simulink model "DiscreteControllerSim"  (R2015b)
settings: Solver=VariableStepAuto  StartTime=0.0  StopTime=t  RelTol=1e-3
values from neighbouring files (symbols this model uses):
  A12 = A(1:3,4:6)    [StateSpace.m]
  C_x = 0.55    [DiscreteController.m]
  C_xdot = -0.17    [DiscreteController.m]
  C_y = 0.55    [DiscreteController.m]
  C_ydot = 0.17    [DiscreteController.m]
  C_z = 0.9    [DiscreteController.m]
  Lobs = (-place(A22',A12',[-20 -25 -30]))'    [StateSpace.m]
  step_x = 1    [DiscreteController.m]
  T = 0.035    [DiscreteController.m]
  x_ref = 1    [plotSim.m]
  x_ref_time = 0.1    [plotSim.m]
  y_ref = 1    [plotSim.m]
  y_ref_time = 5    [plotSim.m]
  z_ref = 1    [plotSim.m]
  z_ref_time = 10    [plotSim.m]
undefined symbols (not defined in the file or in its folder): Fg, Jx, Jy, Jz, kd, kth, L, m, w1_bar, w2_bar, w3_bar, w4_bar
settings Model: Creator=USUARIO  LastModifiedBy=USUARIO

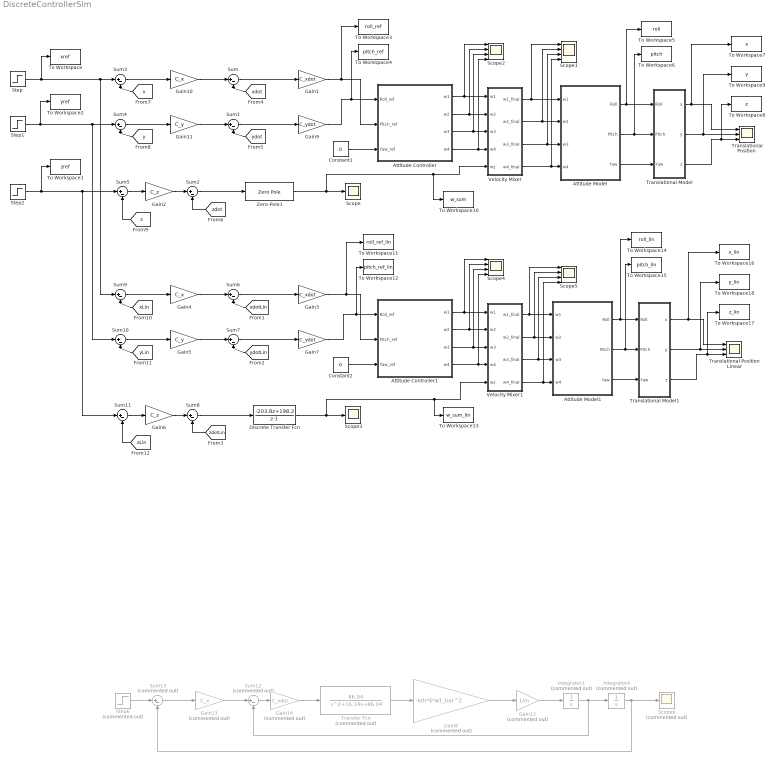
== system DiscreteControllerSim ==
  Attitude Controller : Subsystem
  Attitude Controller1 : Subsystem
  Attitude Model : Subsystem
  Attitude Model1 : Subsystem
  Constant1 : Constant  Value=0
  Constant2 : Constant  Value=0
  Discrete Transfer Fcn : DiscreteTransferFcn  Numerator=[-203.8 198.2]  Denominator=[1 -1]  SampleTime=T
  Gain1 : Gain  Gain=C_xdot
  Gain10 : Gain  Gain=C_x
  Gain11 : Gain  Gain=C_y
  Gain12 : Gain  Commented=on  Gain=1/m
  Gain13 : Gain  Commented=on  Gain=C_x
  Gain14 : Gain  Commented=on  Gain=C_xdot
  Gain2 : Gain  Gain=C_z
  Gain3 : Gain  Gain=C_xdot
  Gain4 : Gain  Gain=C_x
  Gain5 : Gain  Gain=C_y
  Gain6 : Gain  Gain=C_z
  Gain7 : Gain  Gain=C_ydot
  Gain8 : Gain  Commented=on  Gain=-kth*4*w1_bar^2
  Gain9 : Gain  Gain=C_ydot
  Integrator1 : Integrator  Commented=on
  Integrator4 : Integrator  Commented=on
  Scope : Scope
  Scope{1..2,4..5} (4 alike) : Scope  NumInputPorts=4
  Scope3 : Scope
  Scope6 : Scope  Commented=on
  Step : Step  Time=x_ref_time  After=x_ref  SampleTime=0
  Step1 : Step  Time=y_ref_time  After=y_ref  SampleTime=0
  Step2 : Step  Time=z_ref_time  After=z_ref  SampleTime=0
  Step6 : Step  Commented=on  Time=0  After=step_x  SampleTime=0
  Sum{,1..11} (12 alike) : Sum  Inputs=|+-
  Sum12 : Sum  Commented=on  Inputs=|+-
  Sum13 : Sum  Commented=on  Inputs=|+-
  To Workspace : ToWorkspace  VariableName=xref  SaveFormat=Timeseries  SampleTime=-1
  To Workspace1 : ToWorkspace  VariableName=zref  SaveFormat=Timeseries  SampleTime=-1
  To Workspace10 : ToWorkspace  VariableName=w_sum  SaveFormat=Timeseries  SampleTime=-1
  To Workspace11 : ToWorkspace  VariableName=roll_ref_lin  SaveFormat=Timeseries  SampleTime=-1
  To Workspace12 : ToWorkspace  VariableName=pitch_ref_lin  SaveFormat=Timeseries  SampleTime=-1
  To Workspace13 : ToWorkspace  VariableName=w_sum_lin  SaveFormat=Timeseries  SampleTime=-1
  To Workspace14 : ToWorkspace  VariableName=roll_lin  SaveFormat=Timeseries  SampleTime=-1
  To Workspace15 : ToWorkspace  VariableName=pitch_lin  SaveFormat=Timeseries  SampleTime=-1
  To Workspace16 : ToWorkspace  VariableName=x_lin  SaveFormat=Timeseries  SampleTime=-1
  To Workspace17 : ToWorkspace  VariableName=z_lin  SaveFormat=Timeseries  SampleTime=-1
  To Workspace18 : ToWorkspace  VariableName=y_lin  SaveFormat=Timeseries  SampleTime=-1
  To Workspace2 : ToWorkspace  VariableName=yref  SaveFormat=Timeseries  SampleTime=-1
  To Workspace3 : ToWorkspace  VariableName=roll_ref  SaveFormat=Timeseries  SampleTime=-1
  To Workspace4 : ToWorkspace  VariableName=pitch_ref  SaveFormat=Timeseries  SampleTime=-1
  To Workspace5 : ToWorkspace  VariableName=roll  SaveFormat=Timeseries  SampleTime=-1
  To Workspace6 : ToWorkspace  VariableName=pitch  SaveFormat=Timeseries  SampleTime=-1
  To Workspace7 : ToWorkspace  VariableName=x  SaveFormat=Timeseries  SampleTime=-1
  To Workspace8 : ToWorkspace  VariableName=z  SaveFormat=Timeseries  SampleTime=-1
  To Workspace9 : ToWorkspace  VariableName=y  SaveFormat=Timeseries  SampleTime=-1
  Transfer Fcn : TransferFcn  Commented=on  Numerator=[86.04]  Denominator=[1 16.14 86.04]
  Translational Position : Scope  NumInputPorts=3
  Translational Position Linear : Scope  NumInputPorts=3
  Translational Model : Subsystem
  Translational Model1 : Subsystem
  Velocity Mixer : Subsystem
  Velocity Mixer1 : Subsystem
  Zero-Pole1 : ZeroPole  Zeros=[-0.8]  Poles=[0]  Gain=[-200]
  wires:
  Sum/1 -> Gain1/1
  Sum1/1 -> Gain9/1
  Sum2/1 -> Zero-Pole1/1
  [zdot] -> Sum2/2
  [ydot] -> Sum1/2
  [xdot] -> Sum/2
  Gain10/1 -> Sum/1
  Gain11/1 -> Sum1/1
  Constant1/1 -> Attitude Controller/3(Yaw_ref)
  Gain1/1 -> To Workspace3/1, Attitude Controller/2(Pitch_ref)
  Gain9/1 -> To Workspace4/1, Attitude Controller/1(Roll_ref)
  Velocity Mixer/1(w1_final) -> Scope1/1, Attitude Model/1(w1)
  Velocity Mixer/2(w2_final) -> Scope1/2, Attitude Model/2(w2)
  Velocity Mixer/3(w3_final) -> Scope1/3, Attitude Model/3(w3)
  Velocity Mixer/4(w4_final) -> Scope1/4, Attitude Model/4(w4)
  Zero-Pole1/1 -> To Workspace10/1, Velocity Mixer/5(wz), Scope/1
  Attitude Controller/1(w1) -> Velocity Mixer/1(w1), Scope2/1
  Attitude Controller/2(w2) -> Velocity Mixer/2(w2), Scope2/2
  Attitude Controller/3(w3) -> Velocity Mixer/3(w3), Scope2/3
  Attitude Controller/4(w4) -> Velocity Mixer/4(w4), Scope2/4
  Gain2/1 -> Sum2/1
  Attitude Model/1(Roll) -> To Workspace5/1, Translational Model/1(Roll)
  Translational Model/1(x) -> To Workspace7/1, Translational Position/1
  Translational Model/2(y) -> To Workspace9/1, Translational Position/2
  Translational Model/3(z) -> To Workspace8/1, Translational Position/3
  Attitude Model/2(Pitch) -> To Workspace6/1, Translational Model/2(Pitch)
  Sum3/1 -> Gain10/1
  Sum4/1 -> Gain11/1
  [y] -> Sum4/2
  [x] -> Sum3/2
  [z] -> Sum5/2
  Sum5/1 -> Gain2/1
  Attitude Model/3(Yaw) -> Translational Model/3("Yaw ")
  Attitude Model1/1(Roll) -> To Workspace14/1, Translational Model1/1(Roll)
  Translational Model1/1(x) -> To Workspace16/1, Translational Position Linear/1
  Translational Model1/2(y) -> To Workspace18/1, Translational Position Linear/2
  Translational Model1/3(z) -> To Workspace17/1, Translational Position Linear/3
  Sum6/1 -> Gain3/1
  Sum7/1 -> Gain7/1
  Sum8/1 -> Discrete Transfer Fcn/1
  [zdotLin] -> Sum8/2
  [ydotLin] -> Sum7/2
  [xdotLin] -> Sum6/2
  Gain4/1 -> Sum6/1
  Gain5/1 -> Sum7/1
  Constant2/1 -> Attitude Controller1/3(Yaw_ref)
  Attitude Controller1/1(w1) -> Velocity Mixer1/1(w1), Scope4/1
  Attitude Controller1/2(w2) -> Velocity Mixer1/2(w2), Scope4/2
  Attitude Controller1/3(w3) -> Velocity Mixer1/3(w3), Scope4/3
  Attitude Controller1/4(w4) -> Velocity Mixer1/4(w4), Scope4/4
  Gain6/1 -> Sum8/1
  Sum9/1 -> Gain4/1
  Sum10/1 -> Gain5/1
  [yLin] -> Sum10/2
  [xLin] -> Sum9/2
  [zLin] -> Sum11/2
  Step2/1 -> To Workspace1/1, Sum11/1, Sum5/1
  Sum11/1 -> Gain6/1
  Step/1 -> To Workspace/1, Sum9/1, Sum3/1
  Step1/1 -> To Workspace2/1, Sum10/1, Sum4/1
  Velocity Mixer1/1(w1_final) -> Scope5/1, Attitude Model1/1(w1)
  Velocity Mixer1/2(w2_final) -> Scope5/2, Attitude Model1/2(w2)
  Velocity Mixer1/3(w3_final) -> Scope5/3, Attitude Model1/3(w3)
  Velocity Mixer1/4(w4_final) -> Scope5/4, Attitude Model1/4(w4)
  Transfer Fcn/1 -> Gain8/1
  Gain8/1 -> Gain12/1
  Gain12/1 -> Integrator1/1
  Sum12/1 -> Gain14/1
  Integrator1/1 -> Sum12/2, Integrator4/1
  Gain13/1 -> Sum12/1
  Sum13/1 -> Gain13/1
  Integrator4/1 -> Scope6/1, Sum13/2
  Step6/1 -> Sum13/1
  Gain14/1 -> Transfer Fcn/1
  Gain3/1 -> To Workspace11/1, Attitude Controller1/2(Pitch_ref)
  Gain7/1 -> To Workspace12/1, Attitude Controller1/1(Roll_ref)
  Discrete Transfer Fcn/1 -> Velocity Mixer1/5(wz), To Workspace13/1, Scope3/1
  Attitude Model1/2(Pitch) -> To Workspace15/1, Translational Model1/2(Pitch)
  Attitude Model1/3(Yaw) -> Translational Model1/3(Yaw)

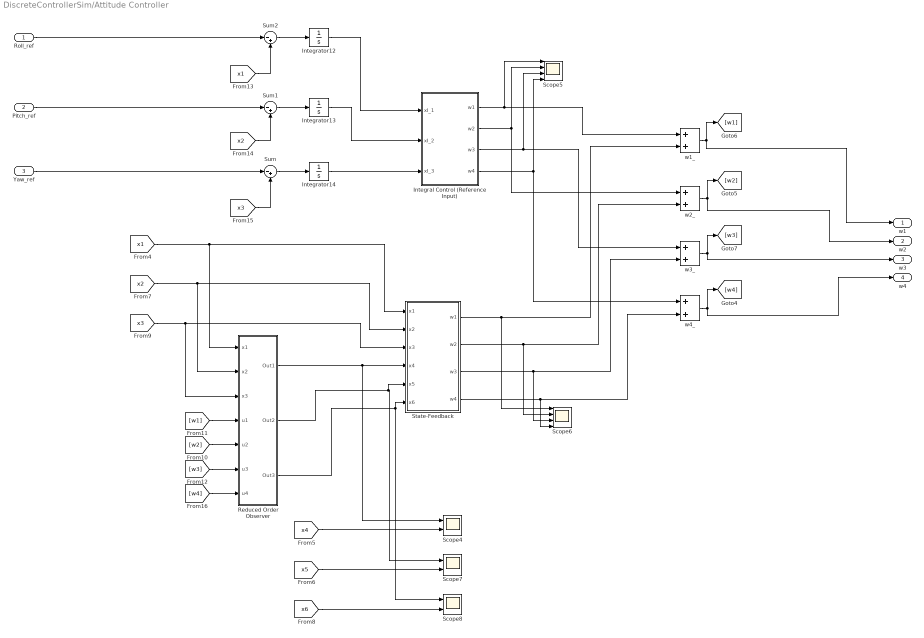
== system DiscreteControllerSim/Attitude Controller ==
  Roll_ref : Inport
  Pitch_ref : Inport  Port=2
  Yaw_ref : Inport  Port=3
  Integral Control (Reference Input) : MATLAB Function  TreatAsAtomicUnit=on
  Integrator12 : Integrator
  Integrator13 : Integrator
  Integrator14 : Integrator
  Reduced Order Observer : Subsystem
  Scope4 : Scope  NumInputPorts=2
  Scope5 : Scope  NumInputPorts=4
  Scope6 : Scope  NumInputPorts=4
  Scope7 : Scope  NumInputPorts=2
  Scope8 : Scope  NumInputPorts=2
  "State-Feedback " : MATLAB Function  TreatAsAtomicUnit=on
  Sum : Sum  Inputs=|-+
  Sum1 : Sum  Inputs=|-+
  Sum2 : Sum  Inputs=|-+
  w1_ : Sum
  w2_ : Sum
  w3_ : Sum
  w4_ : Sum
  w1 : Outport
  w2 : Outport  Port=2
  w3 : Outport  Port=3
  w4 : Outport  Port=4
  wires:
  "State-Feedback "/4(w4) -> w4_/2, Scope6/4
  Roll_ref/1 -> Sum2/1
  [x3] -> Sum/2
  [x1] -> Sum2/2
  Integrator13/1 -> Integral Control (Reference Input)/2(xI_2)
  "State-Feedback "/1(w1) -> w1_/2, Scope6/1
  [w3] -> Reduced Order Observer/6(u3)
  Sum2/1 -> Integrator12/1
  Sum/1 -> Integrator14/1
  [x3] -> "State-Feedback "/3(x3), Reduced Order Observer/3(x3)
  [w2] -> Reduced Order Observer/5(u2)
  Pitch_ref/1 -> Sum1/1
  Integrator14/1 -> Integral Control (Reference Input)/3(xI_3)
  Reduced Order Observer/3(Out3) -> "State-Feedback "/6(x6), Scope8/1
  [x4] -> Scope4/2
  [x6] -> Scope8/2
  "State-Feedback "/2(w2) -> w2_/2, Scope6/2
  Integral Control (Reference Input)/2(w2) -> Scope5/2, w2_/1
  [w4] -> Reduced Order Observer/7(u4)
  Integral Control (Reference Input)/3(w3) -> w3_/1, Scope5/3
  Reduced Order Observer/2(Out2) -> "State-Feedback "/5(x5), Scope7/1
  [x1] -> "State-Feedback "/1(x1), Reduced Order Observer/1(x1)
  [w1] -> Reduced Order Observer/4(u1)
  Integrator12/1 -> Integral Control (Reference Input)/1(xI_1)
  [x2] -> Sum1/2
  Integral Control (Reference Input)/4(w4) -> Scope5/4, w4_/1
  Integral Control (Reference Input)/1(w1) -> w1_/1, Scope5/1
  [x2] -> "State-Feedback "/2(x2), Reduced Order Observer/2(x2)
  Reduced Order Observer/1(Out1) -> "State-Feedback "/4(x4), Scope4/1
  [x5] -> Scope7/2
  Sum1/1 -> Integrator13/1
  Yaw_ref/1 -> Sum/1
  "State-Feedback "/3(w3) -> w3_/2, Scope6/3
  w1_/1 -> w1/1, [w1]
  w4_/1 -> w4/1, [w4]
  w2_/1 -> w2/1, [w2]
  w3_/1 -> w3/1, [w3]

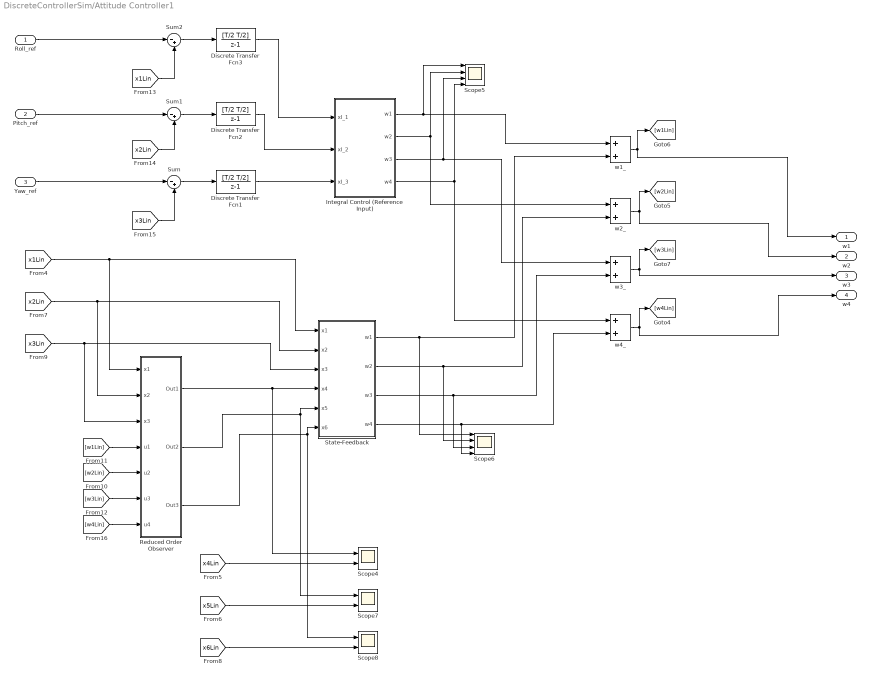
== system DiscreteControllerSim/Attitude Controller1 ==
  Roll_ref : Inport
  Pitch_ref : Inport  Port=2
  Yaw_ref : Inport  Port=3
  Discrete Transfer Fcn1 : DiscreteTransferFcn  Numerator=[T/2 T/2]  Denominator=[1 -1]  SampleTime=T
  Discrete Transfer Fcn2 : DiscreteTransferFcn  Numerator=[T/2 T/2]  Denominator=[1 -1]  SampleTime=T
  Discrete Transfer Fcn3 : DiscreteTransferFcn  Numerator=[T/2 T/2]  Denominator=[1 -1]  SampleTime=T
  Integral Control (Reference Input) : MATLAB Function  TreatAsAtomicUnit=on
  Reduced Order Observer : Subsystem
  Scope4 : Scope  NumInputPorts=2
  Scope5 : Scope  NumInputPorts=4
  Scope6 : Scope  NumInputPorts=4
  Scope7 : Scope  NumInputPorts=2
  Scope8 : Scope  NumInputPorts=2
  "State-Feedback " : MATLAB Function  TreatAsAtomicUnit=on
  Sum : Sum  Inputs=|-+
  Sum1 : Sum  Inputs=|-+
  Sum2 : Sum  Inputs=|-+
  w1_ : Sum
  w2_ : Sum
  w3_ : Sum
  w4_ : Sum
  w1 : Outport
  w2 : Outport  Port=2
  w3 : Outport  Port=3
  w4 : Outport  Port=4
  wires:
  "State-Feedback "/4(w4) -> w4_/2, Scope6/4
  Roll_ref/1 -> Sum2/1
  [x3Lin] -> Sum/2
  [x1Lin] -> Sum2/2
  Discrete Transfer Fcn2/1 -> Integral Control (Reference Input)/2(xI_2)
  "State-Feedback "/1(w1) -> w1_/2, Scope6/1
  [w3Lin] -> Reduced Order Observer/6(u3)
  Sum2/1 -> Discrete Transfer Fcn3/1
  Sum/1 -> Discrete Transfer Fcn1/1
  [x3Lin] -> "State-Feedback "/3(x3), Reduced Order Observer/3(x3)
  [w2Lin] -> Reduced Order Observer/5(u2)
  Pitch_ref/1 -> Sum1/1
  Discrete Transfer Fcn1/1 -> Integral Control (Reference Input)/3(xI_3)
  Reduced Order Observer/3(Out3) -> "State-Feedback "/6(x6), Scope8/1
  [x4Lin] -> Scope4/2
  [x6Lin] -> Scope8/2
  "State-Feedback "/2(w2) -> w2_/2, Scope6/2
  Integral Control (Reference Input)/2(w2) -> Scope5/2, w2_/1
  [w4Lin] -> Reduced Order Observer/7(u4)
  Integral Control (Reference Input)/3(w3) -> w3_/1, Scope5/3
  Reduced Order Observer/2(Out2) -> "State-Feedback "/5(x5), Scope7/1
  [x1Lin] -> "State-Feedback "/1(x1), Reduced Order Observer/1(x1)
  [w1Lin] -> Reduced Order Observer/4(u1)
  Discrete Transfer Fcn3/1 -> Integral Control (Reference Input)/1(xI_1)
  [x2Lin] -> Sum1/2
  Integral Control (Reference Input)/4(w4) -> Scope5/4, w4_/1
  Integral Control (Reference Input)/1(w1) -> w1_/1, Scope5/1
  [x2Lin] -> "State-Feedback "/2(x2), Reduced Order Observer/2(x2)
  Reduced Order Observer/1(Out1) -> "State-Feedback "/4(x4), Scope4/1
  [x5Lin] -> Scope7/2
  Sum1/1 -> Discrete Transfer Fcn2/1
  Yaw_ref/1 -> Sum/1
  "State-Feedback "/3(w3) -> w3_/2, Scope6/3
  w1_/1 -> w1/1, [w1Lin]
  w4_/1 -> w4/1, [w4Lin]
  w2_/1 -> w2/1, [w2Lin]
  w3_/1 -> w3/1, [w3Lin]

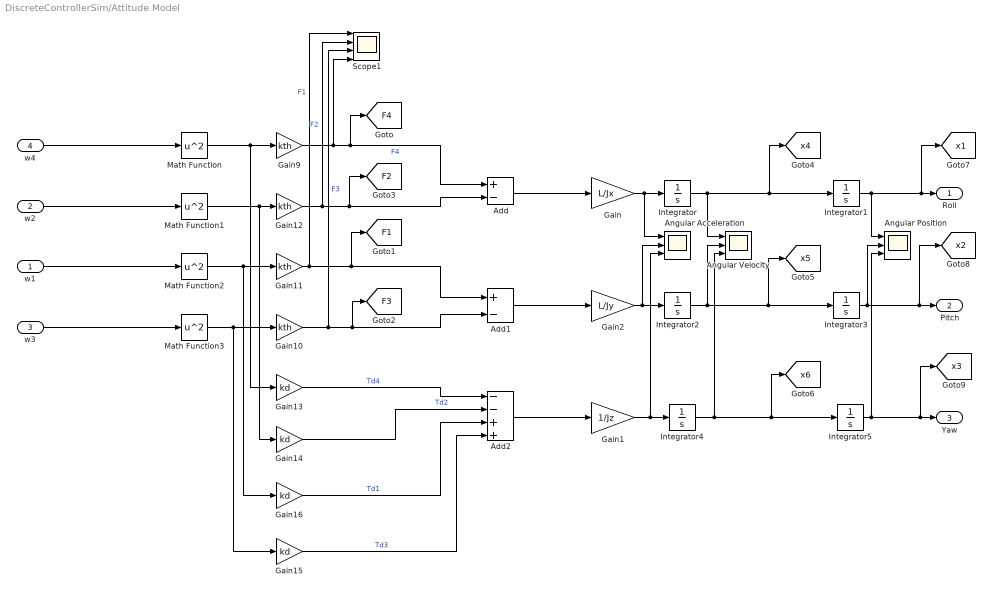
== system DiscreteControllerSim/Attitude Model ==
  w1 : Inport
  w2 : Inport  Port=2
  w3 : Inport  Port=3
  w4 : Inport  Port=4
  Add : Sum  Inputs=+-
  Add1 : Sum  Inputs=+-
  Add2 : Sum  Inputs=--++
  Angular Position : Scope  NumInputPorts=3
  Angular Velocity : Scope  NumInputPorts=3
  Angular Acceleration : Scope  NumInputPorts=3
  Gain : Gain  Gain=L/Jx
  Gain1 : Gain  Gain=1/Jz
  Gain{9..12} (4 alike) : Gain  Gain=kth
  Gain{13..16} (4 alike) : Gain  Gain=kd
  Gain2 : Gain  Gain=L/Jy
  Integrator{,1..5} (6 alike) : Integrator
  Math Function{,1..3} (4 alike) : Math  Operator=square  SaturateOnIntegerOverflow=on
  Scope1 : Scope  NumInputPorts=4
  Roll : Outport
  Pitch : Outport  Port=2
  Yaw : Outport  Port=3
  tag scope: F1=global, F2=global, F3=global, F4=global, x1=global, x2=global, x3=global, x4=global, x5=global, x6=global
  wires:
  Gain2/1 -> Angular Acceleration/2, Integrator2/1
  Add2/1 -> Gain1/1
  Gain9/1 -> Scope1/4, [F4], Add/1  "F4"
  Gain14/1 -> Add2/2  "Td2"
  Gain16/1 -> Add2/3  "Td1"
  Gain/1 -> Angular Acceleration/1, Integrator/1
  Integrator/1 -> Angular Velocity/1, Integrator1/1, [x4]
  Integrator1/1 -> [x1], Roll/1, Angular Position/1
  Integrator4/1 -> Angular Velocity/3, [x6], Integrator5/1
  Add/1 -> Gain/1
  Integrator3/1 -> [x2], Pitch/1, Angular Position/2
  Add1/1 -> Gain2/1
  Integrator5/1 -> Angular Position/3, [x3], Yaw/1
  Gain12/1 -> Scope1/2, [F2], Add/2  "F2"
  Gain10/1 -> [F3], Add1/2, Scope1/3  "F3"
  Gain11/1 -> Scope1/1, [F1], Add1/1  "F1"
  Gain13/1 -> Add2/1  "Td4"
  Gain15/1 -> Add2/4  "Td3"
  Integrator2/1 -> Angular Velocity/2, [x5], Integrator3/1
  Gain1/1 -> Angular Acceleration/3, Integrator4/1
  Math Function3/1 -> Gain15/1, Gain10/1
  Math Function2/1 -> Gain16/1, Gain11/1
  Math Function/1 -> Gain13/1, Gain9/1
  Math Function1/1 -> Gain14/1, Gain12/1
  w1/1 -> Math Function2/1
  w2/1 -> Math Function1/1
  w3/1 -> Math Function3/1
  w4/1 -> Math Function/1

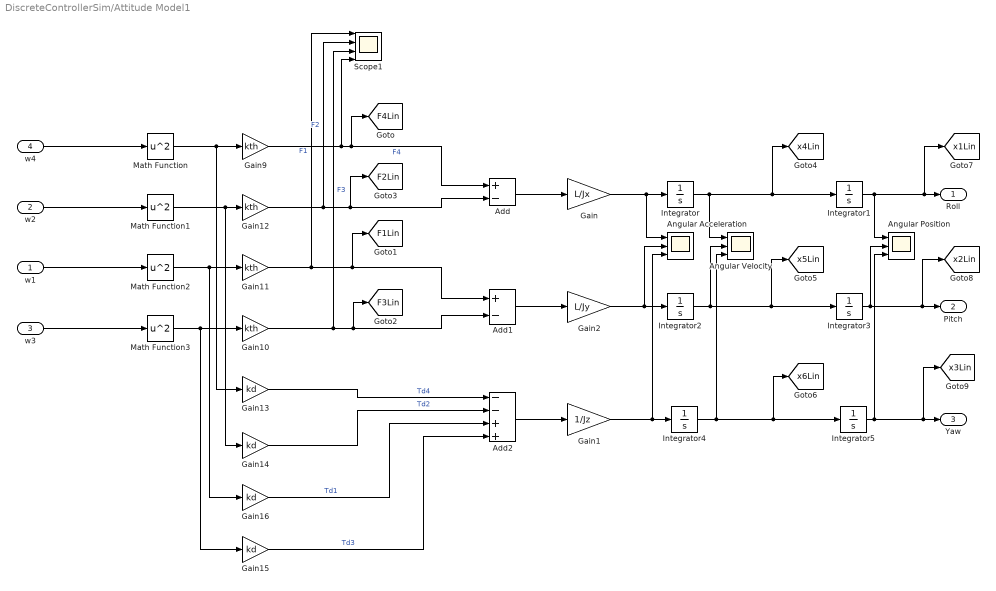
== system DiscreteControllerSim/Attitude Model1 ==
  w1 : Inport
  w2 : Inport  Port=2
  w3 : Inport  Port=3
  w4 : Inport  Port=4
  Add : Sum  Inputs=+-
  Add1 : Sum  Inputs=+-
  Add2 : Sum  Inputs=--++
  Angular Position : Scope  NumInputPorts=3
  Angular Velocity : Scope  NumInputPorts=3
  Angular Acceleration : Scope  NumInputPorts=3
  Gain : Gain  Gain=L/Jx
  Gain1 : Gain  Gain=1/Jz
  Gain{9..12} (4 alike) : Gain  Gain=kth
  Gain{13..16} (4 alike) : Gain  Gain=kd
  Gain2 : Gain  Gain=L/Jy
  Integrator{,1..5} (6 alike) : Integrator
  Math Function{,1..3} (4 alike) : Math  Operator=square  SaturateOnIntegerOverflow=on
  Scope1 : Scope  NumInputPorts=4
  Roll : Outport
  Pitch : Outport  Port=2
  Yaw : Outport  Port=3
  tag scope: F1Lin=global, F2Lin=global, F3Lin=global, F4Lin=global, x1Lin=global, x2Lin=global, x3Lin=global, x4Lin=global, x5Lin=global, x6Lin=global
  wires:
  Gain1/1 -> Integrator4/1, Angular Acceleration/3
  Integrator2/1 -> Integrator3/1, [x5Lin], Angular Velocity/2
  Gain15/1 -> Add2/4  "Td3"
  Gain13/1 -> Add2/1  "Td4"
  Gain11/1 -> Add1/1, [F1Lin], Scope1/1  "F1"
  Gain10/1 -> Scope1/3, Add1/2, [F3Lin]  "F3"
  Gain12/1 -> Scope1/2, Add/2, [F2Lin]  "F2"
  Integrator5/1 -> Yaw/1, [x3Lin], Angular Position/3
  Add1/1 -> Gain2/1
  Integrator3/1 -> Angular Position/2, Pitch/1, [x2Lin]
  Add/1 -> Gain/1
  Integrator4/1 -> Integrator5/1, [x6Lin], Angular Velocity/3
  Integrator1/1 -> Angular Position/1, Roll/1, [x1Lin]
  Integrator/1 -> [x4Lin], Integrator1/1, Angular Velocity/1
  Gain/1 -> Integrator/1, Angular Acceleration/1
  Gain16/1 -> Add2/3  "Td1"
  Gain14/1 -> Add2/2  "Td2"
  Gain9/1 -> Scope1/4, Add/1, [F4Lin]  "F4"
  Add2/1 -> Gain1/1
  Gain2/1 -> Integrator2/1, Angular Acceleration/2
  Math Function3/1 -> Gain15/1, Gain10/1
  Math Function2/1 -> Gain16/1, Gain11/1
  Math Function/1 -> Gain13/1, Gain9/1
  Math Function1/1 -> Gain14/1, Gain12/1
  w1/1 -> Math Function2/1
  w2/1 -> Math Function1/1
  w3/1 -> Math Function3/1
  w4/1 -> Math Function/1

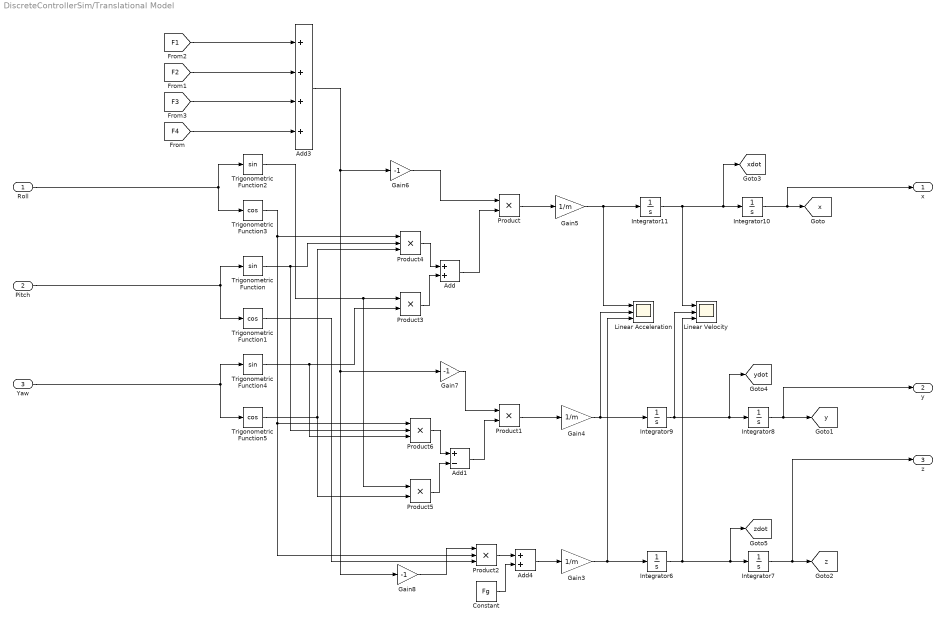
== system DiscreteControllerSim/Translational Model ==
  Roll : Inport
  Pitch : Inport  Port=2
  "Yaw " : Inport  Port=3
  Add : Sum
  Add1 : Sum  Inputs=+-
  Add3 : Sum  Inputs=4
  Add4 : Sum  Inputs=2
  Constant : Constant  Value=Fg
  Gain3 : Gain  Gain=1/m
  Gain4 : Gain  Gain=1/m
  Gain5 : Gain  Gain=1/m
  Gain6 : Gain  Gain=-1
  Gain7 : Gain  Gain=-1
  Gain8 : Gain  Gain=-1
  Integrator{6..11} (6 alike) : Integrator
  Linear Acceleration : Scope  NumInputPorts=3
  Linear Velocity : Scope  NumInputPorts=3
  Product{,1,3,5} (4 alike) : Product
  Product2 : Product  Inputs=3
  Product4 : Product  Inputs=3
  Product6 : Product  Inputs=3
  Trigonometric Function : Trigonometry
  Trigonometric Function1 : Trigonometry  Operator=cos
  Trigonometric Function2 : Trigonometry
  Trigonometric Function3 : Trigonometry  Operator=cos
  Trigonometric Function4 : Trigonometry
  Trigonometric Function5 : Trigonometry  Operator=cos
  x : Outport
  y : Outport  Port=2
  z : Outport  Port=3
  tag scope: x=global, xdot=global, y=global, ydot=global, z=global, zdot=global
  wires:
  Integrator11/1 -> [xdot], Integrator10/1, Linear Velocity/1
  Integrator7/1 -> z/1, [z]
  Gain5/1 -> Integrator11/1, Linear Acceleration/1
  Integrator9/1 -> [ydot], Integrator8/1, Linear Velocity/2
  Integrator10/1 -> [x], x/1
  Integrator8/1 -> y/1, [y]
  [F3] -> Add3/3
  Product/1 -> Gain5/1
  Product1/1 -> Gain4/1
  Gain4/1 -> Integrator9/1, Linear Acceleration/2
  Integrator6/1 -> [zdot], Integrator7/1, Linear Velocity/3
  Gain7/1 -> Product1/1
  Trigonometric Function2/1 -> Product5/1, Product3/1
  Constant/1 -> Add4/2
  [F4] -> Add3/4
  Add3/1 -> Gain8/1, Gain7/1, Gain6/1
  [F2] -> Add3/2
  Trigonometric Function1/1 -> Product2/3
  [F1] -> Add3/1
  Product2/1 -> Add4/1
  Add4/1 -> Gain3/1
  Gain6/1 -> Product/1
  Gain8/1 -> Product2/1
  Trigonometric Function3/1 -> Product4/1, Product6/1, Product2/2
  Gain3/1 -> Integrator6/1, Linear Acceleration/3
  Roll/1 -> Trigonometric Function3/1, Trigonometric Function2/1
  Pitch/1 -> Trigonometric Function/1, Trigonometric Function1/1
  Add/1 -> Product/2
  Product3/1 -> Add/2
  Product4/1 -> Add/1
  "Yaw "/1 -> Trigonometric Function4/1, Trigonometric Function5/1
  Trigonometric Function/1 -> Product6/2, Product4/2
  Trigonometric Function5/1 -> Product4/3, Product5/2
  Trigonometric Function4/1 -> Product6/3, Product3/2
  Product5/1 -> Add1/2
  Product6/1 -> Add1/1
  Add1/1 -> Product1/2

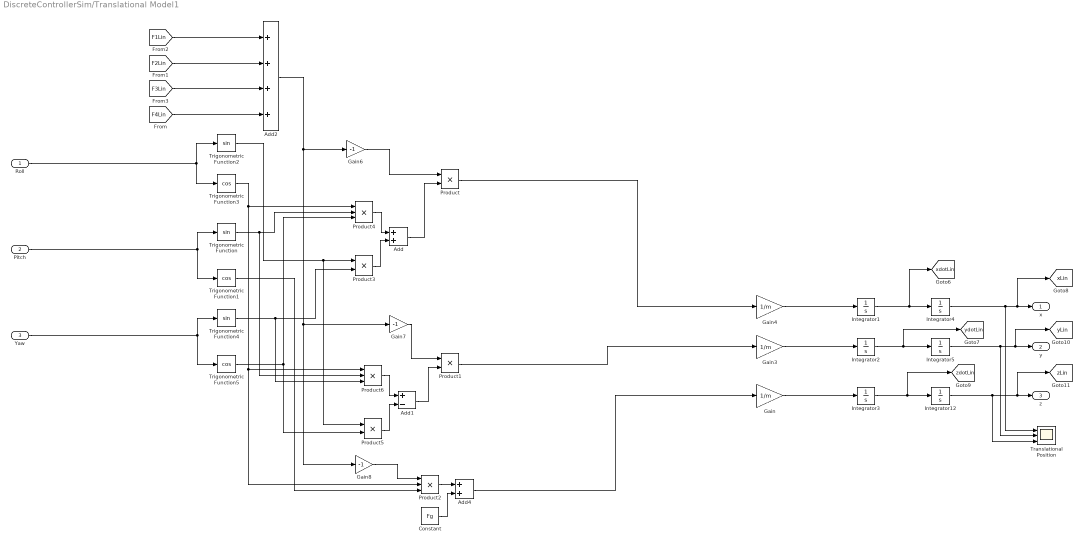
== system DiscreteControllerSim/Translational Model1 ==
  Roll : Inport
  Pitch : Inport  Port=2
  Yaw : Inport  Port=3
  Add : Sum
  Add1 : Sum  Inputs=+-
  Add2 : Sum  Inputs=4
  Add4 : Sum  Inputs=2
  Constant : Constant  Value=Fg
  Gain : Gain  Gain=1/m
  Gain3 : Gain  Gain=1/m
  Gain4 : Gain  Gain=1/m
  Gain6 : Gain  Gain=-1
  Gain7 : Gain  Gain=-1
  Gain8 : Gain  Gain=-1
  Integrator{1..5,12} (6 alike) : Integrator
  Product{,1,3,5} (4 alike) : Product
  Product2 : Product  Inputs=3
  Product4 : Product  Inputs=3
  Product6 : Product  Inputs=3
  Translational Position : Scope  NumInputPorts=3
  Trigonometric Function : Trigonometry
  Trigonometric Function1 : Trigonometry  Operator=cos
  Trigonometric Function2 : Trigonometry
  Trigonometric Function3 : Trigonometry  Operator=cos
  Trigonometric Function4 : Trigonometry
  Trigonometric Function5 : Trigonometry  Operator=cos
  x : Outport
  y : Outport  Port=2
  z : Outport  Port=3
  tag scope: xLin=global, xdotLin=global, yLin=global, ydotLin=global, zLin=global, zdotLin=global
  wires:
  Product/1 -> Gain4/1
  Product1/1 -> Gain3/1
  Integrator1/1 -> [xdotLin], Integrator4/1
  Integrator2/1 -> [ydotLin], Integrator5/1
  Integrator3/1 -> [zdotLin], Integrator12/1
  Integrator4/1 -> Translational Position/1, [xLin], x/1
  Integrator5/1 -> Translational Position/2, [yLin], y/1
  Integrator12/1 -> Translational Position/3, [zLin], z/1
  Gain/1 -> Integrator3/1
  Gain3/1 -> Integrator2/1
  Gain4/1 -> Integrator1/1
  [F3Lin] -> Add2/3
  Gain7/1 -> Product1/1
  Trigonometric Function2/1 -> Product5/1, Product3/1
  Constant/1 -> Add4/2
  [F4Lin] -> Add2/4
  Add2/1 -> Gain8/1, Gain7/1, Gain6/1
  [F2Lin] -> Add2/2
  Trigonometric Function1/1 -> Product2/3
  [F1Lin] -> Add2/1
  Product2/1 -> Add4/1
  Gain6/1 -> Product/1
  Gain8/1 -> Product2/1
  Trigonometric Function3/1 -> Product4/1, Product6/1, Product2/2
  Roll/1 -> Trigonometric Function3/1, Trigonometric Function2/1
  Pitch/1 -> Trigonometric Function/1, Trigonometric Function1/1
  Add/1 -> Product/2
  Product3/1 -> Add/2
  Product4/1 -> Add/1
  Yaw/1 -> Trigonometric Function4/1, Trigonometric Function5/1
  Trigonometric Function/1 -> Product6/2, Product4/2
  Trigonometric Function5/1 -> Product4/3, Product5/2
  Trigonometric Function4/1 -> Product6/3, Product3/2
  Product5/1 -> Add1/2
  Product6/1 -> Add1/1
  Add1/1 -> Product1/2
  Add4/1 -> Gain/1

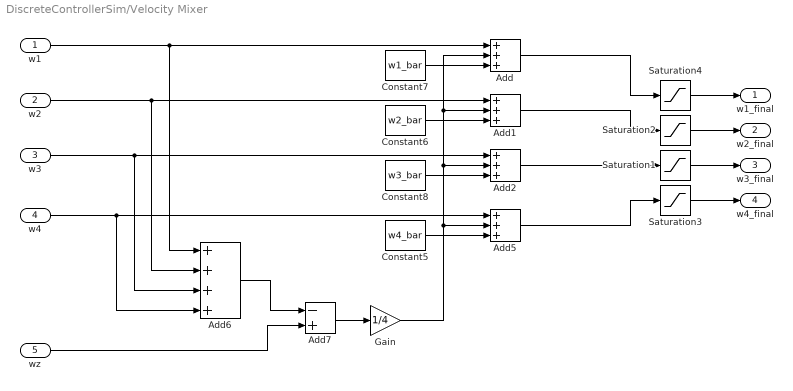
== system DiscreteControllerSim/Velocity Mixer ==
  w1 : Inport
  w2 : Inport  Port=2
  w3 : Inport  Port=3
  w4 : Inport  Port=4
  wz : Inport  Port=5
  Add{,1..2,5} (4 alike) : Sum  Inputs=+++
  Add6 : Sum  Inputs=4
  Add7 : Sum  Inputs=-+
  Constant5 : Constant  Value=w4_bar
  Constant6 : Constant  Value=w2_bar
  Constant7 : Constant  Value=w1_bar
  Constant8 : Constant  Value=w3_bar
  Gain : Gain  Gain=1/4
  Saturation{1..4} (4 alike) : Saturate  UpperLimit=500  LowerLimit=300
  w1_final : Outport
  w2_final : Outport  Port=2
  w3_final : Outport  Port=3
  w4_final : Outport  Port=4
  wires:
  w4/1 -> Add6/4, Add5/1
  Gain/1 -> Add1/2, Add/2, Add2/2, Add5/2
  Add7/1 -> Gain/1
  Add6/1 -> Add7/1
  w2/1 -> Add6/2, Add1/1
  w3/1 -> Add6/3, Add2/1
  wz/1 -> Add7/2
  Add/1 -> Saturation4/1
  Add1/1 -> Saturation2/1
  Add2/1 -> Saturation1/1
  Add5/1 -> Saturation3/1
  w1/1 -> Add/1, Add6/1
  Constant7/1 -> Add/3
  Constant6/1 -> Add1/3
  Constant8/1 -> Add2/3
  Constant5/1 -> Add5/3
  Saturation2/1 -> w2_final/1
  Saturation1/1 -> w3_final/1
  Saturation4/1 -> w1_final/1
  Saturation3/1 -> w4_final/1

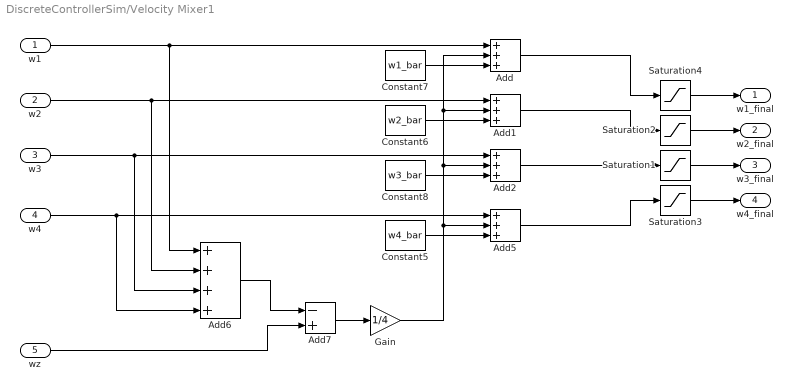
== system DiscreteControllerSim/Velocity Mixer1 ==
  w1 : Inport
  w2 : Inport  Port=2
  w3 : Inport  Port=3
  w4 : Inport  Port=4
  wz : Inport  Port=5
  Add{,1..2,5} (4 alike) : Sum  Inputs=+++
  Add6 : Sum  Inputs=4
  Add7 : Sum  Inputs=-+
  Constant5 : Constant  Value=w4_bar
  Constant6 : Constant  Value=w2_bar
  Constant7 : Constant  Value=w1_bar
  Constant8 : Constant  Value=w3_bar
  Gain : Gain  Gain=1/4
  Saturation{1..4} (4 alike) : Saturate  UpperLimit=500  LowerLimit=300
  w1_final : Outport
  w2_final : Outport  Port=2
  w3_final : Outport  Port=3
  w4_final : Outport  Port=4
  wires:
  w4/1 -> Add6/4, Add5/1
  Gain/1 -> Add1/2, Add/2, Add2/2, Add5/2
  Add7/1 -> Gain/1
  Add6/1 -> Add7/1
  w2/1 -> Add6/2, Add1/1
  w3/1 -> Add6/3, Add2/1
  wz/1 -> Add7/2
  Add/1 -> Saturation4/1
  Add1/1 -> Saturation2/1
  Add2/1 -> Saturation1/1
  Add5/1 -> Saturation3/1
  w1/1 -> Add/1, Add6/1
  Constant7/1 -> Add/3
  Constant6/1 -> Add1/3
  Constant8/1 -> Add2/3
  Constant5/1 -> Add5/3
  Saturation2/1 -> w2_final/1
  Saturation1/1 -> w3_final/1
  Saturation4/1 -> w1_final/1
  Saturation3/1 -> w4_final/1

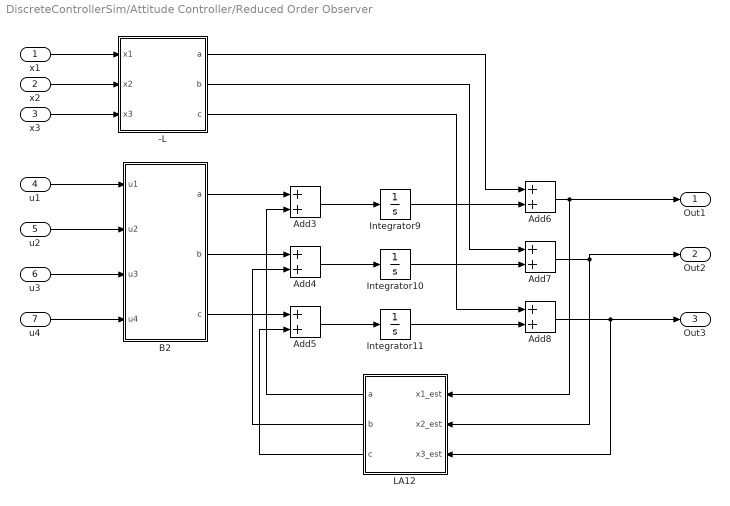
== system DiscreteControllerSim/Attitude Controller/Reduced Order Observer ==
  x1 : Inport
  x2 : Inport  Port=2
  x3 : Inport  Port=3
  u1 : Inport  Port=4
  u2 : Inport  Port=5
  u3 : Inport  Port=6
  u4 : Inport  Port=7
  "-L " : MATLAB Function  TreatAsAtomicUnit=on
  Add{3..8} (6 alike) : Sum  Inputs=2
  B2 : MATLAB Function  TreatAsAtomicUnit=on
  Integrator10 : Integrator
  Integrator11 : Integrator
  Integrator9 : Integrator
  LA12 : MATLAB Function  TreatAsAtomicUnit=on
  Out1 : Outport
  Out2 : Outport  Port=2
  Out3 : Outport  Port=3
  wires:
  Add4/1 -> Integrator10/1
  Add3/1 -> Integrator9/1
  Add5/1 -> Integrator11/1
  u4/1 -> B2/4(u4)
  u2/1 -> B2/2(u2)
  B2/1(a) -> Add3/1
  B2/2(b) -> Add4/1
  B2/3(c) -> Add5/1
  LA12/1(a) -> Add3/2
  LA12/2(b) -> Add4/2
  LA12/3(c) -> Add5/2
  Add6/1 -> LA12/1(x1_est), Out1/1
  Add7/1 -> LA12/2(x2_est), Out2/1
  Add8/1 -> LA12/3(x3_est), Out3/1
  "-L "/3(c) -> Add8/1
  "-L "/1(a) -> Add6/1
  "-L "/2(b) -> Add7/1
  x2/1 -> "-L "/2(x2)
  x3/1 -> "-L "/3(x3)
  x1/1 -> "-L "/1(x1)
  Integrator9/1 -> Add6/2
  Integrator11/1 -> Add8/2
  Integrator10/1 -> Add7/2
  u1/1 -> B2/1(u1)
  u3/1 -> B2/3(u3)

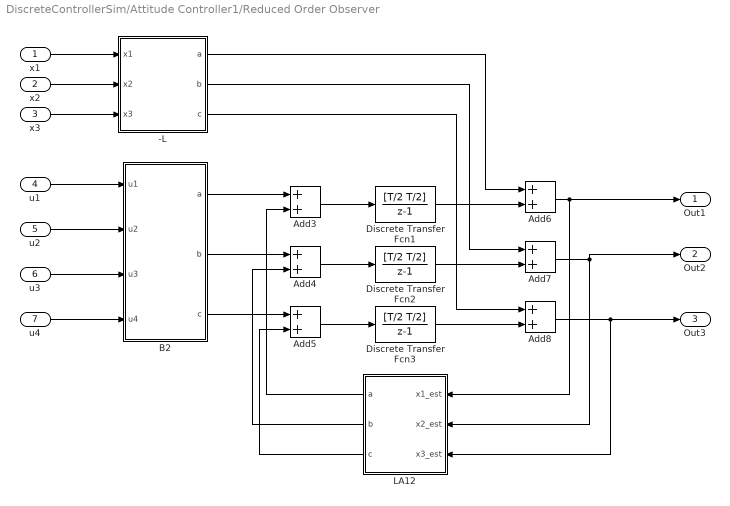
== system DiscreteControllerSim/Attitude Controller1/Reduced Order Observer ==
  x1 : Inport
  x2 : Inport  Port=2
  x3 : Inport  Port=3
  u1 : Inport  Port=4
  u2 : Inport  Port=5
  u3 : Inport  Port=6
  u4 : Inport  Port=7
  "-L " : MATLAB Function  TreatAsAtomicUnit=on
  Add{3..8} (6 alike) : Sum  Inputs=2
  B2 : MATLAB Function  TreatAsAtomicUnit=on
  Discrete Transfer Fcn1 : DiscreteTransferFcn  Numerator=[T/2 T/2]  Denominator=[1 -1]  SampleTime=T
  Discrete Transfer Fcn2 : DiscreteTransferFcn  Numerator=[T/2 T/2]  Denominator=[1 -1]  SampleTime=T
  Discrete Transfer Fcn3 : DiscreteTransferFcn  Numerator=[T/2 T/2]  Denominator=[1 -1]  SampleTime=T
  LA12 : MATLAB Function  TreatAsAtomicUnit=on
  Out1 : Outport
  Out2 : Outport  Port=2
  Out3 : Outport  Port=3
  wires:
  Add4/1 -> Discrete Transfer Fcn2/1
  Add3/1 -> Discrete Transfer Fcn1/1
  Add5/1 -> Discrete Transfer Fcn3/1
  u4/1 -> B2/4(u4)
  u2/1 -> B2/2(u2)
  B2/1(a) -> Add3/1
  B2/2(b) -> Add4/1
  B2/3(c) -> Add5/1
  LA12/1(a) -> Add3/2
  LA12/2(b) -> Add4/2
  LA12/3(c) -> Add5/2
  Add6/1 -> LA12/1(x1_est), Out1/1
  Add7/1 -> LA12/2(x2_est), Out2/1
  Add8/1 -> LA12/3(x3_est), Out3/1
  "-L "/3(c) -> Add8/1
  "-L "/1(a) -> Add6/1
  "-L "/2(b) -> Add7/1
  x2/1 -> "-L "/2(x2)
  x3/1 -> "-L "/3(x3)
  x1/1 -> "-L "/1(x1)
  Discrete Transfer Fcn1/1 -> Add6/2
  Discrete Transfer Fcn3/1 -> Add8/2
  Discrete Transfer Fcn2/1 -> Add7/2
  u1/1 -> B2/1(u1)
  u3/1 -> B2/3(u3)

== matlab function DiscreteControllerSim/Attitude Controller/State-Feedback  ==
  data: x1 input; w1 output; w2 output; w3 output; w4 output; x2 input; x3 input; x4 input; x5 input; x6 input; F parameter
function [w1,w2,w3,w4] = F_matrix(x1, x2, x3, x4, x5, x6, F)
x=[x1;
    x2;
    x3;
    x4;
    x5;
    x6];

w=F*x;

w1=w(1);
w2=w(2);
w3=w(3);
w4=w(4);

== matlab function DiscreteControllerSim/Attitude Controller/Integral Control (Reference Input) ==
  data: xI_1 input; w1 output; w2 output; w3 output; w4 output; xI_2 input; xI_3 input; FI parameter
function [w1,w2,w3,w4] = FI_matrix(xI_1, xI_2, xI_3,FI)
xI=[xI_1;
    xI_2;
    xI_3];

w=FI*xI;

w1=w(1);
w2=w(2);
w3=w(3);
w4=w(4);

== matlab function DiscreteControllerSim/Attitude Controller/Reduced Order Observer/-L  ==
  data: x1 input; a output; b output; c output; x2 input; x3 input; Lobs parameter
function [a,b,c] = minusL_matrix(x1, x2, x3, Lobs)
x=[x1;
    x2;
    x3];

abc=-Lobs*x;

a=abc(1);
b=abc(2);
c=abc(3);

== matlab function DiscreteControllerSim/Attitude Controller/Reduced Order Observer/B2 ==
  data: u1 input; a output; b output; c output; u2 input; u3 input; u4 input; B2 parameter
function [a, b, c] = B2_matrix(u1, u2, u3, u4, B2)
u=[u1;
    u2;
    u3;
    u4];

abc=B2*u;

a=abc(1);
b=abc(2);
c=abc(3);

== matlab function DiscreteControllerSim/Attitude Controller/Reduced Order Observer/LA12 ==
  data: x1_est input; x2_est input; x3_est input; a output; b output; c output; Lobs parameter; A12 parameter
function [a,b,c] = LA12_matrix(x1_est, x2_est, x3_est, Lobs, A12)
x=[x1_est;
    x2_est;
    x3_est];

abc=Lobs*A12*x;

a=abc(1);
b=abc(2);
c=abc(3);

== matlab function DiscreteControllerSim/Attitude Controller1/Integral Control (Reference Input) ==
  data: xI_1 input; w1 output; w2 output; w3 output; w4 output; xI_2 input; xI_3 input; FI parameter
function [w1,w2,w3,w4] = FI_matrix(xI_1, xI_2, xI_3,FI)
xI=[xI_1;
    xI_2;
    xI_3];

w=FI*xI;

w1=w(1);
w2=w(2);
w3=w(3);
w4=w(4);

== matlab function DiscreteControllerSim/Attitude Controller1/Reduced Order Observer/-L  ==
  data: x1 input; a output; b output; c output; x2 input; x3 input; Lobs parameter
function [a,b,c] = minusL_matrix(x1, x2, x3, Lobs)
x=[x1;
    x2;
    x3];

abc=-Lobs*x;

a=abc(1);
b=abc(2);
c=abc(3);

== matlab function DiscreteControllerSim/Attitude Controller1/Reduced Order Observer/B2 ==
  data: u1 input; a output; b output; c output; u2 input; u3 input; u4 input; B2 parameter
function [a, b, c] = B2_matrix(u1, u2, u3, u4, B2)
u=[u1;
    u2;
    u3;
    u4];

abc=B2*u;

a=abc(1);
b=abc(2);
c=abc(3);

== matlab function DiscreteControllerSim/Attitude Controller1/Reduced Order Observer/LA12 ==
  data: x1_est input; x2_est input; x3_est input; a output; b output; c output; Lobs parameter; A12 parameter
function [a,b,c] = LA12_matrix(x1_est, x2_est, x3_est, Lobs, A12)
x=[x1_est;
    x2_est;
    x3_est];

abc=Lobs*A12*x;

a=abc(1);
b=abc(2);
c=abc(3);

== matlab function DiscreteControllerSim/Attitude Controller1/State-Feedback  ==
  data: x1 input; w1 output; w2 output; w3 output; w4 output; x2 input; x3 input; x4 input; x5 input; x6 input; F parameter
function [w1,w2,w3,w4] = F_matrix(x1, x2, x3, x4, x5, x6, F)
x=[x1;
    x2;
    x3;
    x4;
    x5;
    x6];

w=F*x;

w1=w(1);
w2=w(2);
w3=w(3);
w4=w(4);
